simulink model "stewart_platform_dynamics"  (R2019b)
settings: configuration reference "conf_simscape" (kept outside this file)
undefined symbols (not defined in the file): stewart
libraries: nesl_utility x13, sm_lib x4
settings Model: Creator=thomas  LastModifiedBy=thomas
settings ConfigSetRef: SourceName=conf_simscape  SourceLocation=Base Workspace

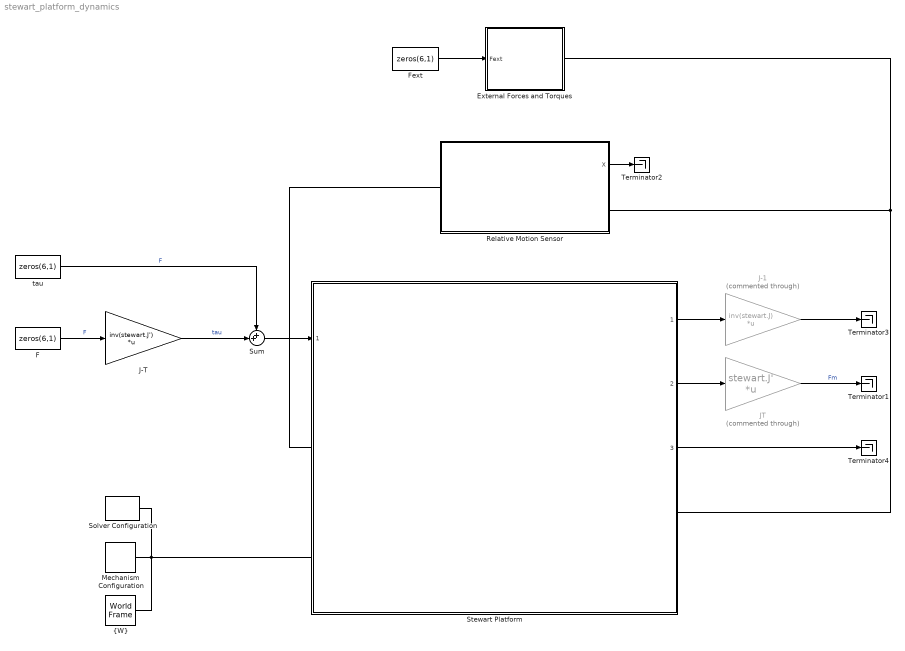
== system stewart_platform_dynamics ==
  External Forces and Torques : Subsystem
  F : Constant  Value=zeros(6,1)
  Fext : Constant  Value=zeros(6,1)
  J-1 : Gain  Commented=through  Gain=inv(stewart.J)  Multiplication=Matrix(K*u)
  J-T : Gain  Gain=inv(stewart.J')  Multiplication=Matrix(K*u)
  JT : Gain  Commented=through  Gain=stewart.J'  Multiplication=Matrix(K*u)
  Mechanism Configuration : sm_lib/Utilities/Mechanism Configuration  UniformGravity=None  GravityVector=[0 0 0]  GravityUnits=m/s^2  LinearizationDelta=0.001
  Relative Motion Sensor : Subsystem
  Solver Configuration : nesl_utility/Solver Configuration  PhysicalDomain=network_engine_domain  SubClassName=solver  LeftPortType=input  RightPortType=generic  Tones=[]  Harmonics=[]  SimulateNoise=off  Profile=off  UseLocalSampling=off  EnableSwitchedLinearOptims=on  FrequencyDomain=off  UseCCode=off  RelTol=0.001  AbsTol=1e-06  MinStep=1e-09  ToWorkspace=off  RevertToSquareIcSolve=off  NumHomotopyIterations=100  PhasorMode=off  PhasorModeNumHarmonics=1  DoDC=off  ResidualTolerance=1e-09  UseLocalSolver=off  LocalSolverChoice=NE_BACKWARD_EULER_ADVANCER  LocalSolverSampleTime=0.001  DoFixedCost=off  MaxNonlinIter=3  MaxModeIter=2  LinearAlgebra=auto  EquationFormulation=NE_TIME_EF  DelaysMemoryBudget=1024  AutomaticFiltering=on  FilteringTimeConstant=0.001  PartitionStorageMethod=AS_NEEDED  PartitionMemoryBudget=1024  PartitionMethod=ROBUST
  Stewart Platform : Subsystem  ReferencedSubsystem=Stewart_Platform
  Sum : Sum  Inputs=++|
  Terminator{1..4} (4 alike) : Terminator
  tau : Constant  Value=zeros(6,1)
  "{W}" : sm_lib/Frames and Transforms/World Frame
  wires:
  F/1 -> J-T/1  "F"
  J-T/1 -> Sum/2  "tau"
  Stewart Platform/2 -> JT/1
  Stewart Platform/1 -> J-1/1
  Fext/1 -> External Forces and Torques/1(Fext)
  Relative Motion Sensor/1(X) -> Terminator2/1
  tau/1 -> Sum/1  "F"
  Sum/1 -> Stewart Platform/1
  Stewart Platform/3 -> Terminator4/1
  J-1/1 -> Terminator3/1
  JT/1 -> Terminator1/1  "Fm"
  connections:
  Stewart Platform/RConn1 -- Relative Motion Sensor/RConn1 -- External Forces and Torques/RConn1
  Mechanism Configuration/RConn1 -- Stewart Platform/LConn2 -- "{W}"/RConn1 -- Solver Configuration/RConn1
  Stewart Platform/LConn1 -- Relative Motion Sensor/LConn1

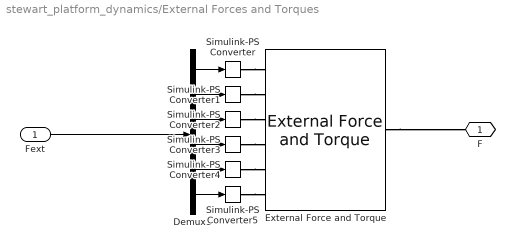
== system stewart_platform_dynamics/External Forces and Torques ==
  Fext : Inport
  Demux1 : Demux  Outputs=6
  External Force and Torque : sm_lib/Forces and Torques/External Force and Torque  ForceResolutionFrame=World  EnableForceX=on  EnableForceY=on  EnableForceZ=on  EnableForce=off  TorqueResolutionFrame=World  EnableTorqueX=on  EnableTorqueY=on  EnableTorqueZ=on  EnableTorque=off
  Simulink-PS Converter{,1..5} (6 alike) : nesl_utility/Simulink-PS Converter  PhysicalDomain=network_engine_domain  SubClassName=ps_input  LeftPortType=input  RightPortType=output  PseudoPeriodic=off  Frequencies=[]  NoiseDistribution=none  NoiseParameters=[]  Unit=1  AffineConversion=off  FilteringAndDerivatives=provide  SimscapeFilterOrder=1  InputFilterTimeConstant=0.001  UdotUserProvided=0
  F : PMIOPort  Side=Right
  wires:
  Demux1/4 -> Simulink-PS Converter3/1
  Demux1/1 -> Simulink-PS Converter/1
  Demux1/6 -> Simulink-PS Converter5/1
  Demux1/2 -> Simulink-PS Converter1/1
  Fext/1 -> Demux1/1
  Demux1/5 -> Simulink-PS Converter4/1
  Demux1/3 -> Simulink-PS Converter2/1
  connections:
  Simulink-PS Converter1/RConn1 -- External Force and Torque/LConn2
  External Force and Torque/RConn1 -- F/RConn1
  Simulink-PS Converter2/RConn1 -- External Force and Torque/LConn3
  Simulink-PS Converter3/RConn1 -- External Force and Torque/LConn4
  Simulink-PS Converter5/RConn1 -- External Force and Torque/LConn6
  Simulink-PS Converter4/RConn1 -- External Force and Torque/LConn5
  Simulink-PS Converter/RConn1 -- External Force and Torque/LConn1

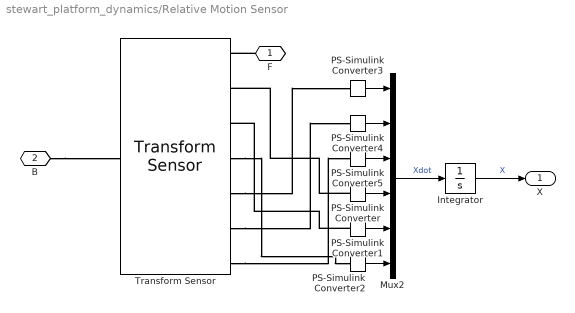
== system stewart_platform_dynamics/Relative Motion Sensor ==
  Integrator : Integrator
  Mux2 : Mux  Inputs=6
  PS-Simulink Converter{,1..5} (6 alike) : nesl_utility/PS-Simulink Converter  PhysicalDomain=network_engine_domain  SubClassName=ps_output  LeftPortType=input  RightPortType=output  PseudoPeriodic=off  Frequencies=[]  Unit=inherit  AffineConversion=off
  Transform Sensor : sm_lib/Frames and Transforms/Transform Sensor  MeasurementFrame=Base  SenseAngle=off  SenseAxis=off  SenseAngle1=off  SenseAngle2=off  SenseAngle3=off  SenseQ=off  SenseR=off  SenseOmegaX=on  SenseOmegaY=on  SenseOmegaZ=on  SenseOmega1=off  SenseOmega2=off  SenseOmega3=off  SenseQDot=off  SenseRDot=off  SenseAlphaX=off  SenseAlphaY=off  SenseAlphaZ=off  SenseAlpha1=off  SenseAlpha2=off  SenseAlpha3=off  SenseQDDot=off  SenseRDDot=off  SenseX=off  SenseY=off  SenseZ=off  SenseRad=off  SenseAzim=off  SenseDist=off  SenseInc=off  SenseXDot=on  SenseYDot=on  SenseZDot=on  SenseRadDot=off  SenseAzimDot=off  SenseDistDot=off  SenseIncDot=off  SenseXDDot=off  SenseYDDot=off  SenseZDDot=off  SenseRadDDot=off  SenseAzimDDot=off  SenseDistDDot=off  SenseIncDDot=off
  F : PMIOPort  Side=Right
  B : PMIOPort  Port=2  Side=Left
  X : Outport
  wires:
  PS-Simulink Converter1/1 -> Mux2/5
  Mux2/1 -> Integrator/1  "Xdot"
  PS-Simulink Converter4/1 -> Mux2/2
  PS-Simulink Converter5/1 -> Mux2/3
  Integrator/1 -> X/1  "X"
  PS-Simulink Converter3/1 -> Mux2/1
  PS-Simulink Converter/1 -> Mux2/4
  PS-Simulink Converter2/1 -> Mux2/6
  connections:
  Transform Sensor/RConn7 -- PS-Simulink Converter5/LConn1
  Transform Sensor/RConn6 -- PS-Simulink Converter4/LConn1
  PS-Simulink Converter/LConn1 -- Transform Sensor/RConn2
  B/RConn1 -- Transform Sensor/LConn1
  F/RConn1 -- Transform Sensor/RConn1
  Transform Sensor/RConn4 -- PS-Simulink Converter2/LConn1
  Transform Sensor/RConn5 -- PS-Simulink Converter3/LConn1
  PS-Simulink Converter1/LConn1 -- Transform Sensor/RConn3
